simulink model "Induction_Motor_from_B_K_Basu_beautified"  (R2019a)
settings: Solver=FixedStepAuto  StartTime=0.0  StopTime=4  FixedStep=1e-6  RelTol=1e-3
undefined symbols (not defined in the file): sigbuilder_block
libraries: powerlib x14
settings Model: Creator=asus  LastModifiedBy=asus

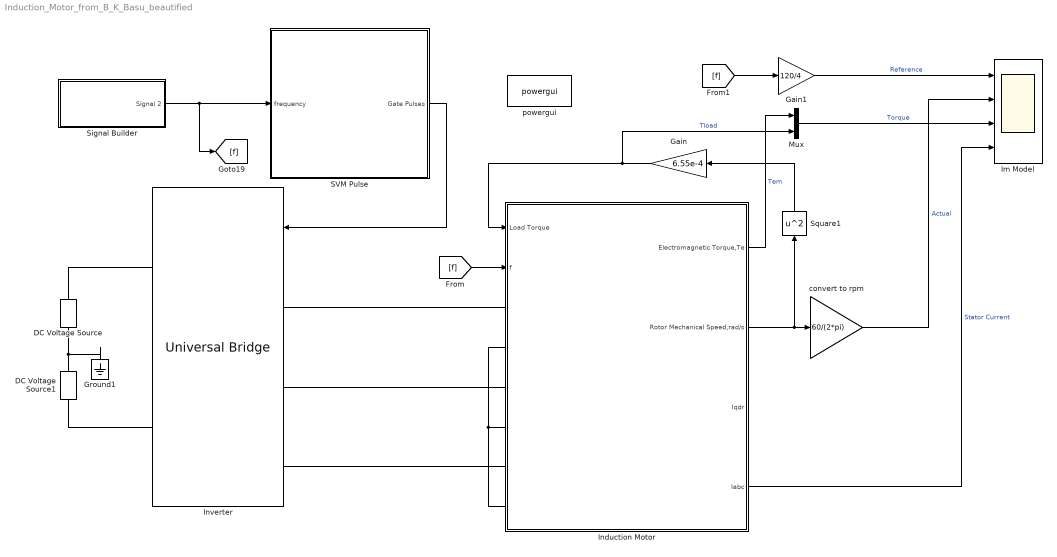
== system Induction_Motor_from_B_K_Basu_beautified ==
  DC Voltage Source : powerlib/Electrical Sources/DC Voltage Source  Amplitude=200  Measurements=None
      settings: SourceProductName=Simscape Electrical
  DC Voltage Source1 : powerlib/Electrical Sources/DC Voltage Source  Amplitude=200  Measurements=None
      settings: SourceProductName=Simscape Electrical
  Gain : Gain  Gain=6.55e-4
  Gain1 : Gain  Gain=120/4
  Ground1 : powerlib/Elements/Ground  LConnTagsString=a
      settings: SourceProductName=Simscape Electrical
  Im Model : Scope  NumInputPorts=4
  Induction Motor : Subsystem  mask{fb=50, Rs=0.603, Rr=0.7, Lls=3.20538e-3, Llr=2.93227e-3, Lm=.0749938, p=4, J=.031, D=.00114}
      mask prompts: fb "Base Frequency. Hz"; Rs "Stator Resistance, Rs"; Rr "Rotor Resistamce, Rr"; Lls "Stator Leakage inductance, Lls"; Llr "Rotor Leakage inductance, Llr"; Lm "Magnetizing Inductance,Lm"; p "Actual Number of Pole,P"; J "Inertia, J"; D "Damping Coefficient,D(Nms)"
      mask help:
      | Frequency is your actual excitation frequency. Base frequency is the maximum frequency for the drive.
      | This are initialized.
      | we=2*pi*f;
      | wb=2*pi*fb;
      | xls=wb*Lls;
      | xlr=wb*Llr;
      | xmeg=wb*Lm;
      | xm=1/(1/xls+1/xlr+1/xmeg);
      mask init:
      | wb=2*pi*fb;
      | xls=wb*Lls;
      | xlr=wb*Llr;
      | xmeg=wb*Lm;
      | xm=1/(1/xls+1/xlr+1/xmeg);
      mask Help:
      | Frequency, f=input from user
      | Base Frequency, fb= input from user
      | Rotor Resistamce= Rr
      | Stator Resistamce= Rs
      | Stator Leakage inductance=Lls
      | Rotor Leakage inductance= Llr
      | Magnetizing Inductance=Lm
      | Actual Number of Pole=p
      | Inertia= J
  Inverter : powerlib/Power Electronics/Universal Bridge  Arms=3  SnubberResistance=1e5  SnubberCapacitance=inf  Device=IGBT / Diodes  Ron=1e-3  Lon=0  ForwardVoltages="[  0  0  ]"  ForwardVoltage=0  GTOparameters=[ 10e-6 , 20e-6 ]  IGBTparameters=[ 1e-6 , 2e-6 ]  Measurements=None  Measurements_2=None  converterType=Rectifier
      settings: SourceProductName=Simscape Electrical
  Mux : Mux  Inputs=2
  SVM Pulse : Subsystem
  Signal Builder : Subsystem  Tag=STV Subsys  LoadFcn=sigbuilder_block('load');  StartFcn=sigbuilder_block('start');  StopFcn=sigbuilder_block('stop');  ClipboardFcn=sigbuilder_block('clipboard');  mask(Sigbuilder block){tuvar=[0:10]}
      mask help: Simulink:masks:SigbuilderBlock_MD
      mask init:
      | if ~strcmp(get_param(bdroot(gcbh),'SimulationStatus'),'stopped') tuvar = sigbuilder_block('maskInit'); end
      settings: CopyFcn=sigbuilder_block('copy');  DeleteFcn=sigbuilder_block('delete');  ModelCloseFcn=sigbuilder_block('modelClose');  PreSaveFcn=sigbuilder_block('preSave');  PauseFcn=sigbuilder_block('pause');  ContinueFcn=sigbuilder_block('continue');  NameChangeFcn=sigbuilder_block('namechange');  OpenFcn=sigbuilder_block('open',[0 30 960 455.4 ]);  CloseFcn=sigbuilder_block('close');
      mask Display: plot(0, 0, 100, 100,[2, 2, 32, 32, 2], [68, 8, 8, 68, 68],[32, 2], [38, 38], [32, 19, 2],[53, 60, 44], [32, 17, 17, 2],[16, 16, 31, 31]);txt = getActiveGroup(gcbh);text(2, 100, txt,'verticalAlignment', 'top');
  Square1 : Math  Operator=square  SaturateOnIntegerOverflow=on
  convert to rpm : Gain  Gain=60/(2*pi)
  powergui : powerlib/powergui  Priority=1  SimulationMode=Discrete  SampleTime=1e-6  frequency=60  Iterations=50  frequencyindice=0  Pbase=100e6  ErrMax=1e-4  UnitsV=kV  UnitsW=MW  buscounter=0  FunctionMessages=off  echomessages=off  EnableUseOfTLC=off  CurrentSourceSwitches=off  DisableSnubberDevices=off  DisableRonSwitches=off  DisableVfSwitches=off  DisplayEquations=off  AutomaticDiscreteSolvers=off  SolverType=Tustin/Backward Euler (TBE)  Interpol=off  ExternalGateDelay=off  methode=off  Ts=100  x0status=blocks  SPID=on  SwTol=0  HookPort=off  NonlinearTolerance=0  nMaxIteration=15  ContinueOnMaxIteration=off  RestoreLinks=warning  ResistiveCurrentMeasurement=off  Frange=[0:2:500]  Ylog=off  Xlog=on  ShowGrid=off  save=off  variable=ZData  structure=0  ZoomFFT=off  StartTime=0.0  cycles=1  DisplayStyle=1  fundamental=60  FreqAxis=off  MaxFrequency=1000  frequencyindicesteady=1  RmsSteady=1  display=off
      settings: SourceProductName=Simscape Electrical
  wires:
  Signal Builder/1(Signal 2) -> [f], SVM Pulse/1(frequency)
  Induction Motor/1(" Electromagnetic Torque,Te ") -> Mux/1  "Tem"
  Induction Motor/2(" Rotor Mechanical Speed,rad/s ") -> Square1/1, convert to rpm/1
  Square1/1 -> Gain/1
  convert to rpm/1 -> Im Model/2  "Actual"
  Gain/1 -> Induction Motor/1(Load Torque), Mux/2  "Tload"
  SVM Pulse/1(Gate Pulses) -> Inverter/1
  [f] -> Induction Motor/2("f ")
  [f] -> Gain1/1
  Gain1/1 -> Im Model/1  "Reference"
  Mux/1 -> Im Model/3  "Torque"
  Induction Motor/4("      Iabc    ") -> Im Model/4  "Stator Current"
  connections:
  Induction Motor/LConn4 -- Induction Motor/LConn2 -- Induction Motor/LConn6
  DC Voltage Source1/RConn1 -- Ground1/LConn1 -- DC Voltage Source/LConn1
  DC Voltage Source1/LConn1 -- Inverter/RConn2
  DC Voltage Source/RConn1 -- Inverter/RConn1
  Inverter/LConn1 -- Induction Motor/LConn1
  Inverter/LConn2 -- Induction Motor/LConn3
  Inverter/LConn3 -- Induction Motor/LConn5

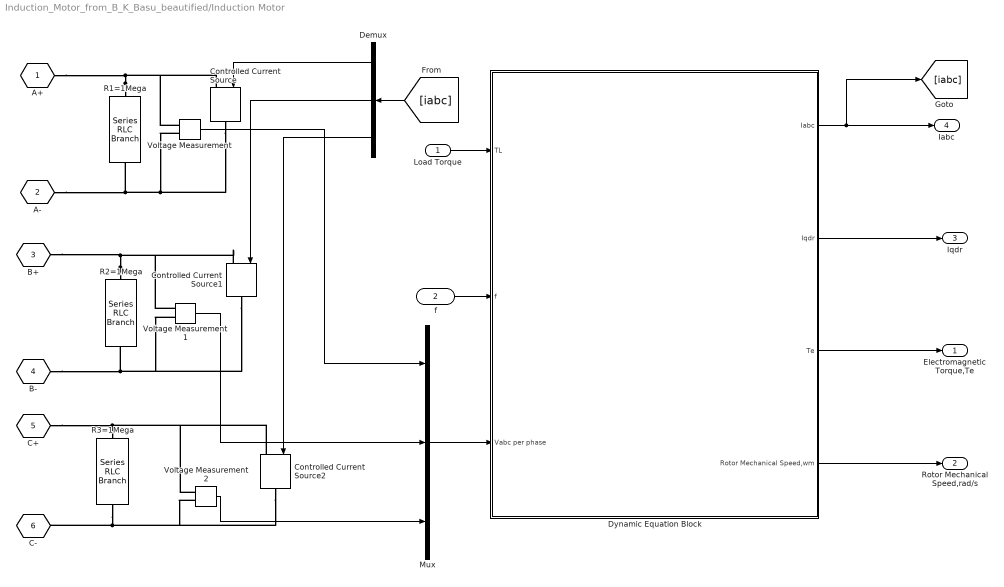
== system Induction_Motor_from_B_K_Basu_beautified/Induction Motor ==
  Load Torque : Inport
  "f " : Inport  Port=2
  Controlled Current Source : powerlib/Electrical Sources/Controlled Current Source  Initialize=on  Source_Type=AC  Amplitude=0  Phase=0  Frequency=0  Measurements=None
      settings: SourceProductName=Simscape Electrical
  Controlled Current Source1 : powerlib/Electrical Sources/Controlled Current Source  Initialize=on  Source_Type=AC  Amplitude=0  Phase=0  Frequency=0  Measurements=None
      settings: SourceProductName=Simscape Electrical
  Controlled Current Source2 : powerlib/Electrical Sources/Controlled Current Source  Initialize=on  Source_Type=AC  Amplitude=0  Phase=0  Frequency=0  Measurements=None
      settings: SourceProductName=Simscape Electrical
  Demux : Demux  Outputs=3
  Dynamic Equation Block : Subsystem
  Mux : Mux  Inputs=3
  R1=1Mega : powerlib/Elements/Series RLC Branch  LConnTagsString=__new0  RConnTagsString=__new0  BranchType=R  Resistance=1e6  Inductance=1e-3  SetiL0=off  InitialCurrent=0  Capacitance=1e-6  Setx0=off  InitialVoltage=0  Measurements=None
      settings: SourceProductName=Simscape Electrical
  R2=1Mega : powerlib/Elements/Series RLC Branch  LConnTagsString=__new0  RConnTagsString=__new0  BranchType=R  Resistance=1e6  Inductance=1e-3  SetiL0=off  InitialCurrent=0  Capacitance=1e-6  Setx0=off  InitialVoltage=0  Measurements=None
      settings: SourceProductName=Simscape Electrical
  R3=1Mega : powerlib/Elements/Series RLC Branch  LConnTagsString=__new0  RConnTagsString=__new0  BranchType=R  Resistance=1e6  Inductance=1e-3  SetiL0=off  InitialCurrent=0  Capacitance=1e-6  Setx0=off  InitialVoltage=0  Measurements=None
      settings: SourceProductName=Simscape Electrical
  Voltage Measurement : powerlib/Measurements/Voltage Measurement  PhasorSimulation=off  OutputType=Complex  PSBequivalent=0
      settings: SourceProductName=Simscape Electrical
  Voltage Measurement1 : powerlib/Measurements/Voltage Measurement  PhasorSimulation=off  OutputType=Complex  PSBequivalent=0
      settings: SourceProductName=Simscape Electrical
  Voltage Measurement2 : powerlib/Measurements/Voltage Measurement  PhasorSimulation=off  OutputType=Complex  PSBequivalent=0
      settings: SourceProductName=Simscape Electrical
  A+ : PMIOPort  Tag=PMCPort  Side=Left
  A- : PMIOPort  Tag=PMCPort  Port=2  Side=Left
  B+ : PMIOPort  Tag=PMCPort  Port=3  Side=Left
  B- : PMIOPort  Tag=PMCPort  Port=4  Side=Left
  C+ : PMIOPort  Tag=PMCPort  Port=5  Side=Left
  C- : PMIOPort  Tag=PMCPort  Port=6  Side=Left
  " Electromagnetic Torque,Te " : Outport
  " Rotor Mechanical Speed,rad/s " : Outport  Port=2
  " Iqdr     " : Outport  Port=3
  "      Iabc    " : Outport  Port=4
  wires:
  Dynamic Equation Block/4("Rotor Mechanical Speed,wm ") -> " Rotor Mechanical Speed,rad/s "/1
  Voltage Measurement/1 -> Mux/1
  Load Torque/1 -> Dynamic Equation Block/1(TL)
  Voltage Measurement1/1 -> Mux/2
  Voltage Measurement2/1 -> Mux/3
  Mux/1 -> Dynamic Equation Block/3(Vabc per phase)
  Dynamic Equation Block/3(Te) -> " Electromagnetic Torque,Te "/1
  Dynamic Equation Block/1(Iabc) -> [iabc], "      Iabc    "/1
  Dynamic Equation Block/2("Iqdr ") -> " Iqdr     "/1
  [iabc] -> Demux/1
  Demux/1 -> Controlled Current Source/1
  Demux/2 -> Controlled Current Source1/1
  Demux/3 -> Controlled Current Source2/1
  "f "/1 -> Dynamic Equation Block/2(f)
  connections:
  Controlled Current Source1/RConn1 -- Voltage Measurement1/LConn2 -- B-/RConn1 -- R2=1Mega/RConn1
  R2=1Mega/LConn1 -- Controlled Current Source1/LConn1 -- Voltage Measurement1/LConn1 -- B+/RConn1
  R3=1Mega/LConn1 -- Controlled Current Source2/LConn1 -- Voltage Measurement2/LConn1 -- C+/RConn1
  R3=1Mega/RConn1 -- Controlled Current Source2/RConn1 -- Voltage Measurement2/LConn2 -- C-/RConn1
  R1=1Mega/LConn1 -- Voltage Measurement/LConn1 -- Controlled Current Source/LConn1 -- A+/RConn1
  Voltage Measurement/LConn2 -- R1=1Mega/RConn1 -- A-/RConn1 -- Controlled Current Source/RConn1

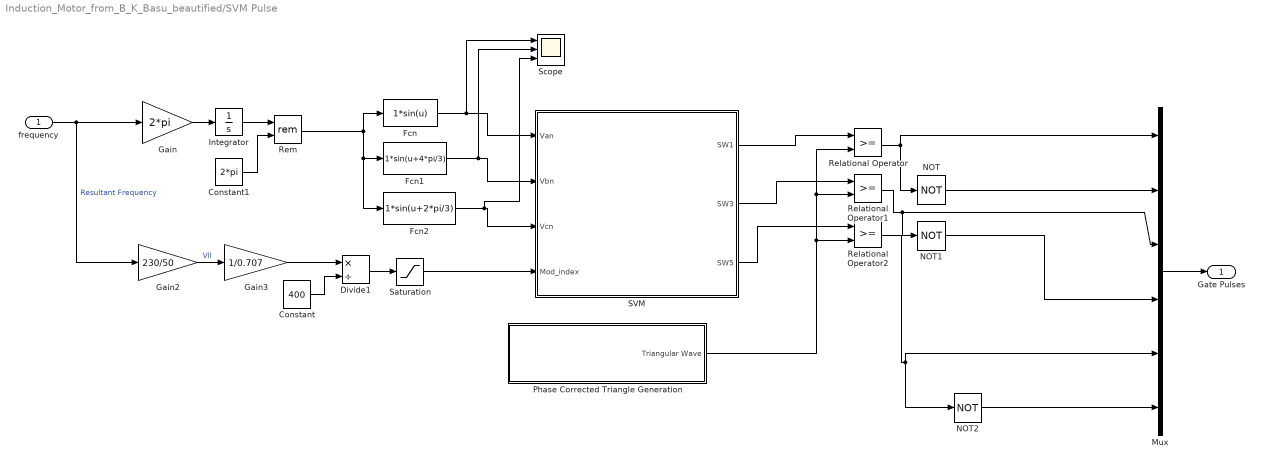
== system Induction_Motor_from_B_K_Basu_beautified/SVM Pulse ==
  frequency : Inport
  Constant : Constant  Value=400
  Constant1 : Constant  Value=2*pi
  Divide1 : Product  Inputs=*/
  Fcn : Fcn  Expr=1*sin(u)
  Fcn1 : Fcn  Expr=1*sin(u+4*pi/3)
  Fcn2 : Fcn  Expr=1*sin(u+2*pi/3)
  Gain : Gain  Gain=2*pi
  Gain2 : Gain  Gain=230/50
  Gain3 : Gain  Gain=1/0.707
  Integrator : Integrator
  Mux : Mux  Inputs=6
  NOT : Logic  Operator=NOT  IconShape=distinctive  AllPortsSameDT=off  OutDataTypeStr=boolean
  NOT1 : Logic  Operator=NOT  IconShape=distinctive  AllPortsSameDT=off  OutDataTypeStr=boolean
  NOT2 : Logic  Operator=NOT  IconShape=distinctive  AllPortsSameDT=off  OutDataTypeStr=boolean
  Phase Corrected Triangle Generation : Subsystem
  Relational Operator : RelationalOperator  OutDataTypeStr=boolean  RndMeth=Nearest
  Relational Operator1 : RelationalOperator  OutDataTypeStr=boolean  RndMeth=Nearest
  Relational Operator2 : RelationalOperator  OutDataTypeStr=boolean  RndMeth=Nearest
  Rem : Math  Operator=rem  SaturateOnIntegerOverflow=on
  SVM : Subsystem
  Saturation : Saturate  UpperLimit=1  LowerLimit=0
  Scope : Scope  NumInputPorts=3
  Gate Pulses : Outport
  wires:
  Phase Corrected Triangle Generation/1(Triangular Wave) -> Relational Operator/2, Relational Operator1/2, Relational Operator2/2
  SVM/3(SW5) -> Relational Operator2/1
  NOT/1 -> Mux/2
  Relational Operator2/1 -> Mux/5, NOT2/1
  Relational Operator1/1 -> NOT1/1, Mux/3
  SVM/1(SW1) -> Relational Operator/1
  SVM/2(SW3) -> Relational Operator1/1
  NOT2/1 -> Mux/6
  Saturation/1 -> SVM/4(Mod_index)
  Relational Operator/1 -> Mux/1, NOT/1
  NOT1/1 -> Mux/4
  Mux/1 -> Gate Pulses/1
  Rem/1 -> Fcn/1, Fcn2/1, Fcn1/1
  Fcn/1 -> Scope/1, SVM/1(Van)
  Fcn1/1 -> Scope/2, SVM/2(Vbn)
  Fcn2/1 -> Scope/3, SVM/3(Vcn)
  Divide1/1 -> Saturation/1
  Gain3/1 -> Divide1/1
  Gain2/1 -> Gain3/1  "Vll"
  frequency/1 -> Gain/1, Gain2/1  "Resultant Frequency"
  Constant/1 -> Divide1/2
  Gain/1 -> Integrator/1
  Integrator/1 -> Rem/1
  Constant1/1 -> Rem/2

== system Induction_Motor_from_B_K_Basu_beautified/Signal Builder ==
  Demux : Demux  Tag=STV Demux  Outputs=1
  FromWs : FromWorkspace  Tag=STV FromWs  VariableName=tuvar  SampleTime=0
      SigBuilderData=|
      | common.afterFinalStr = 'Extrapolate'
      | common.sampleTime = 0
      | dataSet.timeRange = [0 10]
      | dataSet.name = 'Group 1'
      | sbobj.Groups.Name = 'Group 1'
      | sbobj.Groups.Signals.Name = 'Signal 2'
      | sbobj.Groups.Signals.XData = [0 2 3 3 3.5 3.5 4 4 5 10]
      | sbobj.Groups.Signals.YData = [5 50 25 20 20 30 30 10 10 40]
  Signal 2 : Outport  Tag=STV Outport
  wires:
  FromWs/1 -> Demux/1
  Demux/1 -> Signal 2/1

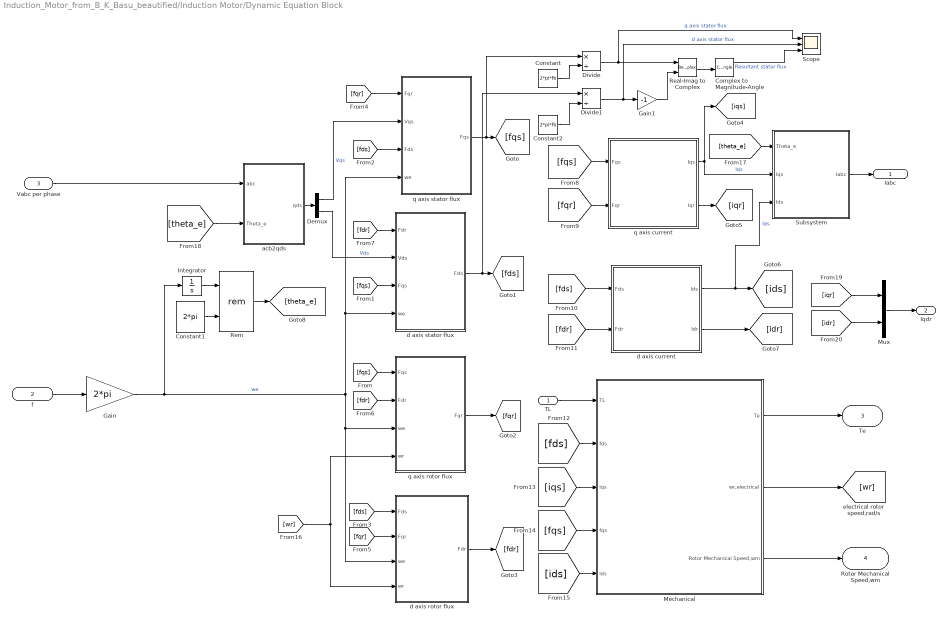
== system Induction_Motor_from_B_K_Basu_beautified/Induction Motor/Dynamic Equation Block ==
  TL : Inport
  f : Inport  Port=2
  Vabc per phase : Inport  Port=3
  Complex to Magnitude-Angle : ComplexToMagnitudeAngle
  Constant : Constant  Value=2*pi*fb
  Constant1 : Constant  Value=2*pi
  Constant2 : Constant  Value=2*pi*fb
  Demux : Demux  Outputs=2
  Divide : Product  Inputs=*/
  Divide1 : Product  Inputs=*/
  Gain : Gain  Gain=2*pi
  Gain1 : Gain  Gain=-1
  Integrator : Integrator
  Mechanical : Subsystem
  Mux : Mux  Inputs=2
  Real-Imag to Complex : RealImagToComplex
  Rem : Math  Operator=rem  SaturateOnIntegerOverflow=on
  Scope : Scope  NumInputPorts=3
  Subsystem : Subsystem
  acb2qds : Subsystem
  d axis current : Subsystem
  d axis rotor flux : Subsystem
  d axis stator flux : Subsystem
  q axis current : Subsystem
  q axis rotor flux : Subsystem
  "q axis stator flux " : Subsystem
  Iabc : Outport
  "Iqdr " : Outport  Port=2
  Te : Outport  Port=3
  "Rotor Mechanical Speed,wm " : Outport  Port=4
  wires:
  "q axis stator flux "/1(Fqs) -> Divide/1, [fqs]
  [fqr] -> "q axis stator flux "/1(Fqr)
  Gain/1 -> d axis rotor flux/3("we "), q axis rotor flux/3("we "), d axis stator flux/4(we), "q axis stator flux "/4(we), Integrator/1  "we"
  [fds] -> "q axis stator flux "/3(Fds)
  [wr] -> d axis rotor flux/4(wr), q axis rotor flux/4(wr)
  Demux/2 -> d axis stator flux/2(Vds)  "Vds"
  d axis rotor flux/1(Fdr) -> [fdr]
  [fds] -> d axis rotor flux/1("Fds  ")
  q axis current/2(Iqr) -> [iqr]
  [fds] -> d axis current/1(Fds)
  [fdr] -> d axis current/2(Fdr)
  [fqs] -> q axis current/1(Fqs)
  q axis current/1(Iqs) -> [iqs], Subsystem/2(Iqs)  "Iqs"
  d axis stator flux/1(Fds) -> Divide1/1, [fds]
  [fqr] -> q axis current/2(Fqr)
  q axis rotor flux/1(Fqr) -> [fqr]
  [fdr] -> d axis stator flux/1("Fdr ")
  [fqs] -> q axis rotor flux/1("Fqs  ")
  [fdr] -> q axis rotor flux/2("Fdr ")
  [fqs] -> d axis stator flux/3("Fqs ")
  [fqr] -> d axis rotor flux/2("Fqr  ")
  d axis current/1(Ids) -> [ids], Subsystem/3(Ids)  "Ids"
  Demux/1 -> "q axis stator flux "/2(Vqs)  "Vqs"
  d axis current/2(Idr) -> [idr]
  acb2qds/1(qds) -> Demux/1
  TL/1 -> Mechanical/1(TL)
  Mechanical/1(Te) -> Te/1
  Mechanical/2(wr,electrical) -> [wr]
  Mechanical/3("Rotor Mechanical Speed,wm ") -> "Rotor Mechanical Speed,wm "/1
  [fds] -> Mechanical/2(fds)
  [iqs] -> Mechanical/3(iqs)
  [fqs] -> Mechanical/4(fqs)
  [ids] -> Mechanical/5(ids)
  Vabc per phase/1 -> acb2qds/1(abc)
  Integrator/1 -> Rem/1
  Constant1/1 -> Rem/2
  Rem/1 -> [theta_e]
  Subsystem/1(Iabc) -> Iabc/1
  [theta_e] -> Subsystem/1(Theta_e)
  [theta_e] -> acb2qds/2(Theta_e)
  [iqr] -> Mux/1
  [idr] -> Mux/2
  Mux/1 -> "Iqdr "/1
  f/1 -> Gain/1
  Constant/1 -> Divide/2
  Constant2/1 -> Divide1/2
  Divide1/1 -> Scope/2, Gain1/1  "d axis stator flux"
  Divide/1 -> Scope/1, Real-Imag to Complex/1  "q axis stator flux"
  Gain1/1 -> Real-Imag to Complex/2
  Real-Imag to Complex/1 -> Complex to Magnitude-Angle/1
  Complex to Magnitude-Angle/1 -> Scope/3  "Resultant stator flux"

== system Induction_Motor_from_B_K_Basu_beautified/SVM Pulse/Phase Corrected Triangle Generation ==
  Constant : Constant
  Gain : Gain  Gain=2*5000
  Integrator : Integrator
  Pulse Generator : DiscretePulseGenerator  PulseType=Time based  Amplitude=2  Period=1/5000  PulseWidth=50
  Sum : Sum  Inputs=|+-
  Triangular Wave : Outport
  wires:
  Gain/1 -> Triangular Wave/1
  Pulse Generator/1 -> Sum/1
  Sum/1 -> Integrator/1
  Integrator/1 -> Gain/1
  Constant/1 -> Sum/2

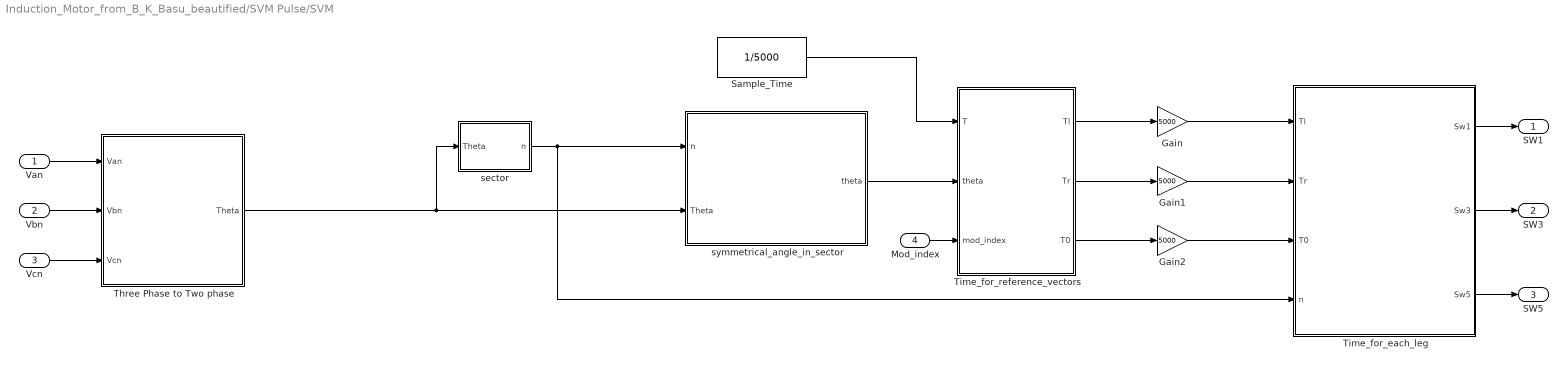
== system Induction_Motor_from_B_K_Basu_beautified/SVM Pulse/SVM ==
  Van : Inport
  Vbn : Inport  Port=2
  Vcn : Inport  Port=3
  Mod_index : Inport  Port=4
  Gain : Gain  Gain=5000
  Gain1 : Gain  Gain=5000
  Gain2 : Gain  Gain=5000
  Sample_Time : Constant  Value=1/5000
  "Three Phase to Two phase " : MATLAB Function  TreatAsAtomicUnit=on
  Time_for_each_leg : MATLAB Function  TreatAsAtomicUnit=on
  Time_for_reference_vectors : MATLAB Function  TreatAsAtomicUnit=on
  "sector " : MATLAB Function  TreatAsAtomicUnit=on
  symmetrical_angle_in_sector : MATLAB Function  TreatAsAtomicUnit=on
  SW1 : Outport
  SW3 : Outport  Port=2
  SW5 : Outport  Port=3
  wires:
  Sample_Time/1 -> Time_for_reference_vectors/1(T)
  Time_for_reference_vectors/2(Tr) -> Gain1/1
  Time_for_reference_vectors/1(Tl) -> Gain/1
  Time_for_reference_vectors/3(T0) -> Gain2/1
  symmetrical_angle_in_sector/1(theta) -> Time_for_reference_vectors/2(theta)
  "Three Phase to Two phase "/1(Theta) -> symmetrical_angle_in_sector/2(Theta), "sector "/1(Theta)
  Vbn/1 -> "Three Phase to Two phase "/2(Vbn)
  Vcn/1 -> "Three Phase to Two phase "/3(Vcn)
  Van/1 -> "Three Phase to Two phase "/1(Van)
  Gain/1 -> Time_for_each_leg/1(Tl)
  Gain1/1 -> Time_for_each_leg/2(Tr)
  Gain2/1 -> Time_for_each_leg/3(T0)
  "sector "/1(n) -> Time_for_each_leg/4(n), symmetrical_angle_in_sector/1(n)
  Time_for_each_leg/1(Sw1) -> SW1/1
  Time_for_each_leg/2(Sw3) -> SW3/1
  Time_for_each_leg/3(Sw5) -> SW5/1
  Mod_index/1 -> Time_for_reference_vectors/3(mod_index)

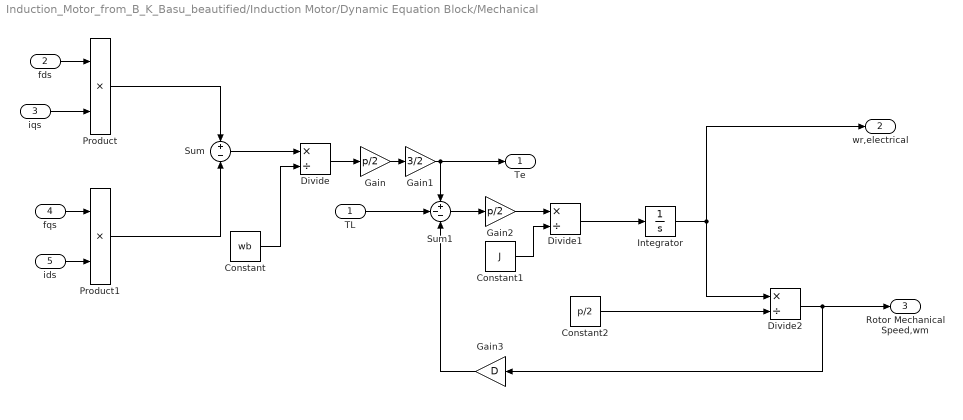
== system Induction_Motor_from_B_K_Basu_beautified/Induction Motor/Dynamic Equation Block/Mechanical ==
  TL : Inport
  fds : Inport  Port=2
  iqs : Inport  Port=3
  fqs : Inport  Port=4
  ids : Inport  Port=5
  Constant : Constant  Value=wb
  Constant1 : Constant  Value=J
  Constant2 : Constant  Value=p/2
  Divide : Product  Inputs=*/
  Divide1 : Product  Inputs=*/
  Divide2 : Product  Inputs=*/
  Gain : Gain  Gain=p/2
  Gain1 : Gain  Gain=3/2
  Gain2 : Gain  Gain=p/2
  Gain3 : Gain  Gain=D
  Integrator : Integrator
  Product : Product
  Product1 : Product
  Sum : Sum  Inputs=+-
  Sum1 : Sum  Inputs=+--
  Te : Outport
  wr,electrical : Outport  Port=2
  "Rotor Mechanical Speed,wm " : Outport  Port=3
  wires:
  Sum1/1 -> Gain2/1
  Product/1 -> Sum/1
  Divide1/1 -> Integrator/1
  Constant2/1 -> Divide2/2
  Constant1/1 -> Divide1/2
  Sum/1 -> Divide/1
  Gain1/1 -> Te/1, Sum1/1
  TL/1 -> Sum1/2
  Divide2/1 -> Gain3/1, "Rotor Mechanical Speed,wm "/1
  Gain/1 -> Gain1/1
  Constant/1 -> Divide/2
  Gain2/1 -> Divide1/1
  Product1/1 -> Sum/2
  Divide/1 -> Gain/1
  fds/1 -> Product/1
  ids/1 -> Product1/2
  fqs/1 -> Product1/1
  iqs/1 -> Product/2
  Integrator/1 -> Divide2/1, wr,electrical/1
  Gain3/1 -> Sum1/3

== system Induction_Motor_from_B_K_Basu_beautified/Induction Motor/Dynamic Equation Block/Subsystem ==
  Theta_e : Inport
  Iqs : Inport  Port=2
  Ids : Inport  Port=3
  Fcn : Fcn  Expr=(u(2)*cos(u(1)))+(u(3)*sin(u(1)))
  Fcn1 : Fcn  Expr=(-u(2)*sin(u(1)))+(u(3)*cos(u(1)))
  Fcn2 : Fcn  Expr=u(1)
  Fcn3 : Fcn  Expr=(-u(1)*1/2)+(-sqrt(3)/2*u(2))
  Fcn4 : Fcn  Expr=(-u(1)*1/2)+(sqrt(3)/2*u(2))
  Mux : Mux  Inputs=3
  Mux1 : Mux  Inputs=2
  Mux2 : Mux  Inputs=3
  Iabc : Outport
  wires:
  Fcn3/1 -> Mux2/2
  Fcn/1 -> Mux1/1  "Iqs"
  Mux1/1 -> Fcn4/1, Fcn3/1, Fcn2/1
  Mux/1 -> Fcn1/1, Fcn/1
  Fcn1/1 -> Mux1/2  "Ids"
  Iqs/1 -> Mux/2
  Fcn2/1 -> Mux2/1
  Fcn4/1 -> Mux2/3
  Mux2/1 -> Iabc/1
  Theta_e/1 -> Mux/1
  Ids/1 -> Mux/3

== system Induction_Motor_from_B_K_Basu_beautified/Induction Motor/Dynamic Equation Block/acb2qds ==
  abc : Inport
  Theta_e : Inport  Port=2
  Fcn : Fcn  Expr=u(1)
  Fcn1 : Fcn  Expr=(-u(2)+u(3))/sqrt(3)
  Fcn2 : Fcn  Expr=(u(1)*cos(u(3)))-(u(2)*sin(u(3)))
  Fcn3 : Fcn  Expr=(u(1)*sin(u(3)))+(u(2)*cos(u(3)))
  Mux1 : Mux  Inputs=2
  Mux2 : Mux  Inputs=3
  qds : Outport
  wires:
  Fcn1/1 -> Mux2/2  "Vdstator"
  abc/1 -> Fcn1/1, Fcn/1
  Mux2/1 -> Fcn3/1, Fcn2/1
  Theta_e/1 -> Mux2/3
  Fcn2/1 -> Mux1/1  "Vqs"
  Fcn3/1 -> Mux1/2  "Vds"
  Mux1/1 -> qds/1
  Fcn/1 -> Mux2/1  "Vqstator"

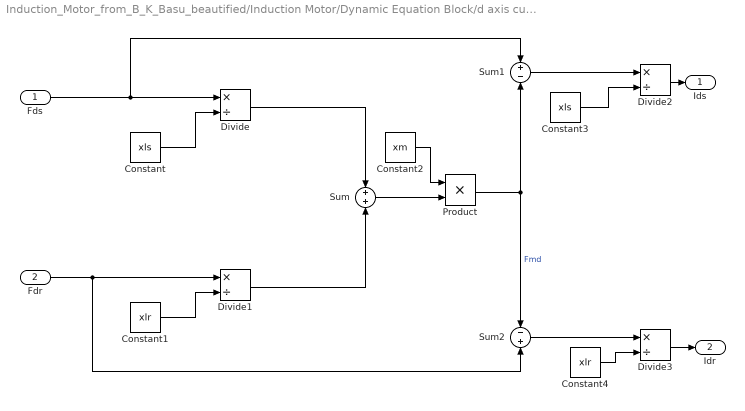
== system Induction_Motor_from_B_K_Basu_beautified/Induction Motor/Dynamic Equation Block/d axis current ==
  Fds : Inport
  Fdr : Inport  Port=2
  Constant : Constant  Value=xls
  Constant1 : Constant  Value=xlr
  Constant2 : Constant  Value=xm
  Constant3 : Constant  Value=xls
  Constant4 : Constant  Value=xlr
  Divide{,1..3} (4 alike) : Product  Inputs=*/
  Product : Product
  Sum : Sum
  Sum1 : Sum  Inputs=+-
  Sum2 : Sum  Inputs=-+
  Ids : Outport
  Idr : Outport  Port=2
  wires:
  Fdr/1 -> Sum2/2, Divide1/1
  Constant2/1 -> Product/1
  Product/1 -> Sum2/1, Sum1/2  "Fmd"
  Constant/1 -> Divide/2
  Sum/1 -> Product/2
  Divide1/1 -> Sum/2
  Constant1/1 -> Divide1/2
  Fds/1 -> Sum1/1, Divide/1
  Divide/1 -> Sum/1
  Sum1/1 -> Divide2/1
  Constant3/1 -> Divide2/2
  Divide2/1 -> Ids/1
  Sum2/1 -> Divide3/1
  Constant4/1 -> Divide3/2
  Divide3/1 -> Idr/1

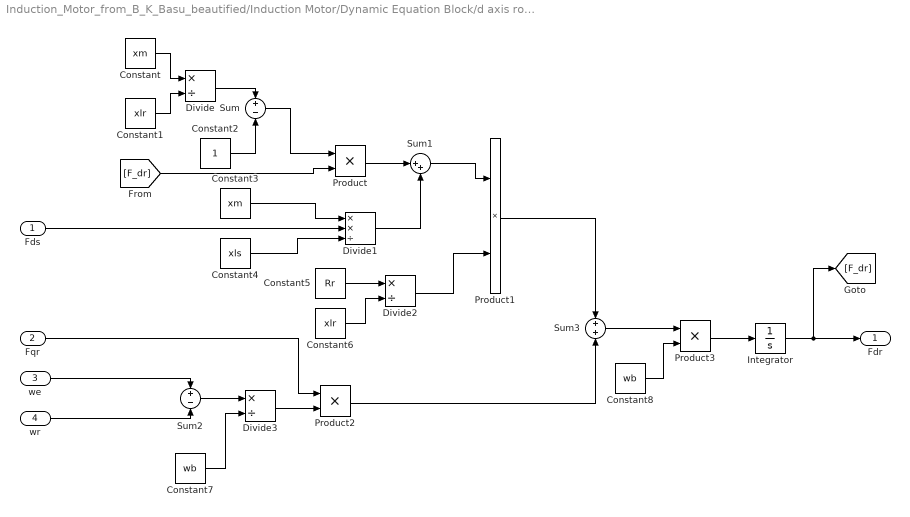
== system Induction_Motor_from_B_K_Basu_beautified/Induction Motor/Dynamic Equation Block/d axis rotor flux ==
  "Fds  " : Inport
  "Fqr  " : Inport  Port=2
  "we " : Inport  Port=3
  wr : Inport  Port=4
  Constant : Constant  Value=xm
  Constant1 : Constant  Value=xlr
  Constant2 : Constant
  Constant3 : Constant  Value=xm
  Constant4 : Constant  Value=xls
  Constant5 : Constant  Value=Rr
  Constant6 : Constant  Value=xlr
  Constant7 : Constant  Value=wb
  Constant8 : Constant  Value=wb
  Divide : Product  Inputs=*/
  Divide1 : Product  Inputs=**/
  Divide2 : Product  Inputs=*/
  Divide3 : Product  Inputs=*/
  Integrator : Integrator
  Product{,1..3} (4 alike) : Product
  Sum : Sum  Inputs=+-
  Sum1 : Sum  Inputs=|++
  Sum2 : Sum  Inputs=+-
  Sum3 : Sum
  Fdr : Outport
  wires:
  Constant2/1 -> Sum/2
  Sum/1 -> Product/1
  Constant/1 -> Divide/1
  Constant3/1 -> Divide1/1
  Sum3/1 -> Product3/1
  "Fds  "/1 -> Divide1/2
  Constant4/1 -> Divide1/3
  [F_dr] -> Product/2
  Divide1/1 -> Sum1/2
  Constant1/1 -> Divide/2
  Product3/1 -> Integrator/1
  Divide/1 -> Sum/1
  Constant5/1 -> Divide2/1
  Constant7/1 -> Divide3/2
  wr/1 -> Sum2/2
  Constant8/1 -> Product3/2
  Product2/1 -> Sum3/2
  "Fqr  "/1 -> Product2/1
  Product/1 -> Sum1/1
  Sum1/1 -> Product1/1
  "we "/1 -> Sum2/1
  Integrator/1 -> [F_dr], Fdr/1
  Sum2/1 -> Divide3/1
  Product1/1 -> Sum3/1
  Divide3/1 -> Product2/2
  Divide2/1 -> Product1/2
  Constant6/1 -> Divide2/2

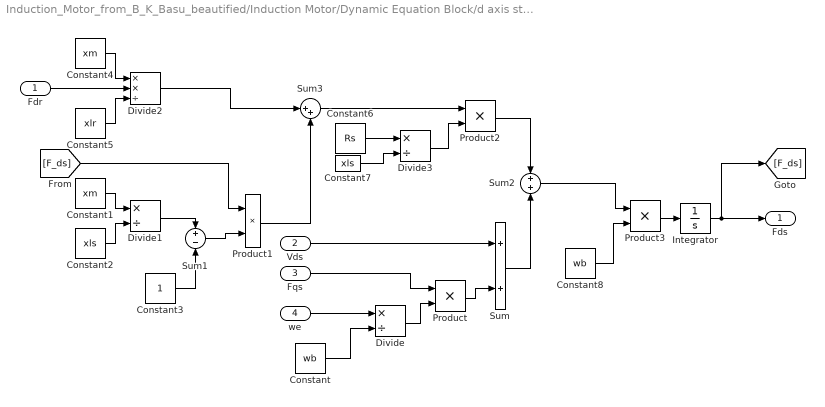
== system Induction_Motor_from_B_K_Basu_beautified/Induction Motor/Dynamic Equation Block/d axis stator flux ==
  "Fdr " : Inport
  Vds : Inport  Port=2
  "Fqs " : Inport  Port=3
  we : Inport  Port=4
  Constant : Constant  Value=wb
  Constant1 : Constant  Value=xm
  Constant2 : Constant  Value=xls
  Constant3 : Constant
  Constant4 : Constant  Value=xm
  Constant5 : Constant  Value=xlr
  Constant6 : Constant  Value=Rs
  Constant7 : Constant  Value=xls
  Constant8 : Constant  Value=wb
  Divide : Product  Inputs=*/
  Divide1 : Product  Inputs=*/
  Divide2 : Product  Inputs=**/
  Divide3 : Product  Inputs=*/
  Integrator : Integrator
  Product{,1..3} (4 alike) : Product
  Sum : Sum
  Sum1 : Sum  Inputs=+-
  Sum2 : Sum
  Sum3 : Sum  Inputs=|++
  Fds : Outport
  wires:
  Constant8/1 -> Product3/2
  "Fdr "/1 -> Divide2/2
  Product2/1 -> Sum2/1
  Vds/1 -> Sum/1
  Divide3/1 -> Product2/2
  Constant7/1 -> Divide3/2
  Constant6/1 -> Divide3/1
  Sum3/1 -> Product2/1
  Product1/1 -> Sum3/2
  Divide2/1 -> Sum3/1
  Constant2/1 -> Divide1/2
  Sum/1 -> Sum2/2
  Constant1/1 -> Divide1/1
  we/1 -> Divide/1
  Product/1 -> Sum/2
  Constant3/1 -> Sum1/2
  Sum1/1 -> Product1/2
  "Fqs "/1 -> Product/1
  Constant/1 -> Divide/2
  Constant5/1 -> Divide2/3
  Divide/1 -> Product/2
  Sum2/1 -> Product3/1
  Divide1/1 -> Sum1/1
  [F_ds] -> Product1/1
  Constant4/1 -> Divide2/1
  Product3/1 -> Integrator/1
  Integrator/1 -> Fds/1, [F_ds]

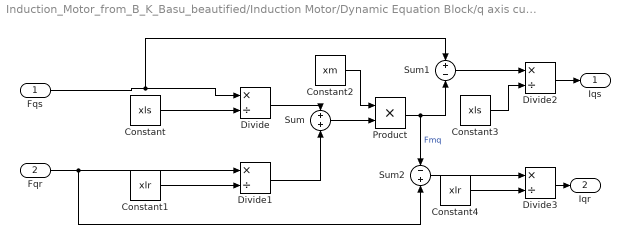
== system Induction_Motor_from_B_K_Basu_beautified/Induction Motor/Dynamic Equation Block/q axis current ==
  Fqs : Inport
  Fqr : Inport  Port=2
  Constant : Constant  Value=xls
  Constant1 : Constant  Value=xlr
  Constant2 : Constant  Value=xm
  Constant3 : Constant  Value=xls
  Constant4 : Constant  Value=xlr
  Divide{,1..3} (4 alike) : Product  Inputs=*/
  Product : Product
  Sum : Sum
  Sum1 : Sum  Inputs=+-
  Sum2 : Sum  Inputs=-+
  Iqs : Outport
  Iqr : Outport  Port=2
  wires:
  Divide/1 -> Sum/1
  Fqs/1 -> Sum1/1, Divide/1
  Constant1/1 -> Divide1/2
  Divide1/1 -> Sum/2
  Sum/1 -> Product/2
  Constant/1 -> Divide/2
  Constant2/1 -> Product/1
  Fqr/1 -> Sum2/2, Divide1/1
  Product/1 -> Sum1/2, Sum2/1  "Fmq"
  Sum1/1 -> Divide2/1
  Constant3/1 -> Divide2/2
  Divide2/1 -> Iqs/1
  Sum2/1 -> Divide3/1
  Constant4/1 -> Divide3/2
  Divide3/1 -> Iqr/1

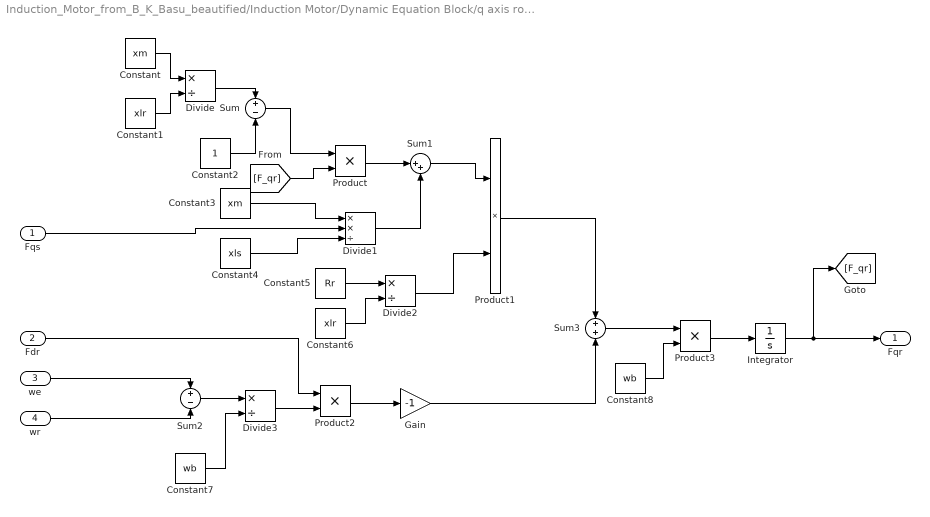
== system Induction_Motor_from_B_K_Basu_beautified/Induction Motor/Dynamic Equation Block/q axis rotor flux ==
  "Fqs  " : Inport
  "Fdr " : Inport  Port=2
  "we " : Inport  Port=3
  wr : Inport  Port=4
  Constant : Constant  Value=xm
  Constant1 : Constant  Value=xlr
  Constant2 : Constant
  Constant3 : Constant  Value=xm
  Constant4 : Constant  Value=xls
  Constant5 : Constant  Value=Rr
  Constant6 : Constant  Value=xlr
  Constant7 : Constant  Value=wb
  Constant8 : Constant  Value=wb
  Divide : Product  Inputs=*/
  Divide1 : Product  Inputs=**/
  Divide2 : Product  Inputs=*/
  Divide3 : Product  Inputs=*/
  Gain : Gain  Gain=-1
  Integrator : Integrator
  Product{,1..3} (4 alike) : Product
  Sum : Sum  Inputs=+-
  Sum1 : Sum  Inputs=|++
  Sum2 : Sum  Inputs=+-
  Sum3 : Sum
  Fqr : Outport
  wires:
  Constant6/1 -> Divide2/2
  Divide2/1 -> Product1/2
  Divide3/1 -> Product2/2
  Product1/1 -> Sum3/1
  Sum2/1 -> Divide3/1
  Integrator/1 -> Fqr/1, [F_qr]
  "we "/1 -> Sum2/1
  Sum1/1 -> Product1/1
  Product2/1 -> Gain/1
  Product/1 -> Sum1/1
  "Fdr "/1 -> Product2/1
  Gain/1 -> Sum3/2
  Constant8/1 -> Product3/2
  wr/1 -> Sum2/2
  Constant7/1 -> Divide3/2
  Constant5/1 -> Divide2/1
  Divide/1 -> Sum/1
  Product3/1 -> Integrator/1
  Constant1/1 -> Divide/2
  Divide1/1 -> Sum1/2
  [F_qr] -> Product/2
  Constant4/1 -> Divide1/3
  "Fqs  "/1 -> Divide1/2
  Sum3/1 -> Product3/1
  Constant3/1 -> Divide1/1
  Constant/1 -> Divide/1
  Sum/1 -> Product/1
  Constant2/1 -> Sum/2

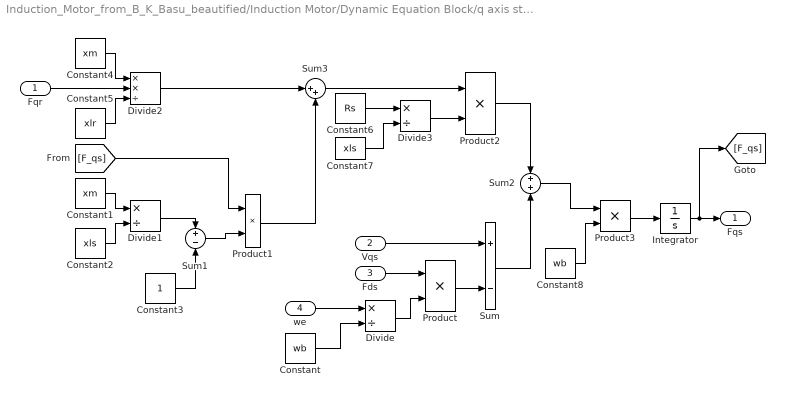
== system Induction_Motor_from_B_K_Basu_beautified/Induction Motor/Dynamic Equation Block/q axis stator flux  ==
  Fqr : Inport
  Vqs : Inport  Port=2
  Fds : Inport  Port=3
  we : Inport  Port=4
  Constant : Constant  Value=wb
  Constant1 : Constant  Value=xm
  Constant2 : Constant  Value=xls
  Constant3 : Constant
  Constant4 : Constant  Value=xm
  Constant5 : Constant  Value=xlr
  Constant6 : Constant  Value=Rs
  Constant7 : Constant  Value=xls
  Constant8 : Constant  Value=wb
  Divide : Product  Inputs=*/
  Divide1 : Product  Inputs=*/
  Divide2 : Product  Inputs=**/
  Divide3 : Product  Inputs=*/
  Integrator : Integrator
  Product{,1..3} (4 alike) : Product
  Sum : Sum  Inputs=+-
  Sum1 : Sum  Inputs=+-
  Sum2 : Sum
  Sum3 : Sum  Inputs=|++
  Fqs : Outport
  wires:
  Constant4/1 -> Divide2/1
  [F_qs] -> Product1/1
  Divide1/1 -> Sum1/1
  Sum2/1 -> Product3/1
  Divide/1 -> Product/2
  Constant5/1 -> Divide2/3
  Constant/1 -> Divide/2
  Fds/1 -> Product/1
  Sum1/1 -> Product1/2
  Constant3/1 -> Sum1/2
  Product/1 -> Sum/2
  we/1 -> Divide/1
  Constant1/1 -> Divide1/1
  Sum/1 -> Sum2/2
  Constant2/1 -> Divide1/2
  Divide2/1 -> Sum3/1
  Product1/1 -> Sum3/2
  Sum3/1 -> Product2/1
  Constant6/1 -> Divide3/1
  Constant7/1 -> Divide3/2
  Divide3/1 -> Product2/2
  Vqs/1 -> Sum/1
  Product2/1 -> Sum2/1
  Fqr/1 -> Divide2/2
  Constant8/1 -> Product3/2
  Product3/1 -> Integrator/1
  Integrator/1 -> Fqs/1, [F_qs]

== matlab function Induction_Motor_from_B_K_Basu_beautified/SVM Pulse/SVM/sector  ==
  data: Theta input; n output
function n = sector(Theta)
%#codegen
n=0;
if (Theta<=pi/3) && (Theta >0)
    n=1;
end
if (Theta<=2*pi/3) && (Theta >pi/3)
    n=2;
end
if (Theta<=pi) && (Theta >2*pi/3)
    n=3;
end
if (Theta<=-2*pi/3) && (Theta >-pi)
    n=4;
end
if (Theta<=-pi/3) && (Theta >-2*pi/3)
    n=5;
end
if (Theta<=0) && (Theta >-pi/3)
    n=6;
end

== matlab function Induction_Motor_from_B_K_Basu_beautified/SVM Pulse/SVM/Three Phase to Two phase  ==
  data: Van input; Vbn input; Vcn input; Theta output
function Theta  = three_to_two_phase(Van,Vbn,Vcn)
%#codegen
Valpha= Van-Vbn/2-Vcn/2;
Vbeta = sqrt(3)/2*(Vbn-Vcn);
Theta = atan2(Vbeta,Valpha);

== matlab function Induction_Motor_from_B_K_Basu_beautified/SVM Pulse/SVM/symmetrical_angle_in_sector ==
  data: n input; Theta input; theta output
function theta = symmetrical_angle_in_sector(n,Theta)
%#codegen
theta=0;
if (n==1)
    theta=Theta;
end
if (n==2)
    theta=Theta-pi/3;
end
if (n==3)
    theta=Theta-2*pi/3;
end
if (n==6)
    theta=pi/3+Theta;
end
if (n==5)
    theta=2*pi/3+Theta;
end
if (n==4)
    theta=pi+Theta;
end

== matlab function Induction_Motor_from_B_K_Basu_beautified/SVM Pulse/SVM/Time_for_reference_vectors ==
  data: Tl output; T input; theta input; Tr output; T0 output; mod_index input
function [Tl,Tr,T0]= Time_for_reference_vectors(T,theta,mod_index)
%#codegen
%a=Vr/Vdc;

%Tr=T*a*(sin(pi/3-theta)/sin(pi/3));
Tr=T*mod_index*sin(pi/3-theta);
% Tl=T*a*sin(theta)/sin(pi/3);
Tl=T*mod_index*sin(theta);
T0=T-Tl-Tr;

== matlab function Induction_Motor_from_B_K_Basu_beautified/SVM Pulse/SVM/Time_for_each_leg ==
  data: Tl input; Sw1 output; Tr input; T0 input; n input; Sw3 output; Sw5 output
function [Sw1,Sw3,Sw5]= Time_for_each_leg(Tl,Tr,T0,n)

%#codegen
Sw1=0;
Sw3=0;
Sw5=0;
if (n==1)
Sw1=Tl+Tr+T0/2;
Sw3=Tl+T0/2;
Sw5=T0/2;
end
if (n==2)
Sw1=Tr+T0/2;
Sw3=Tl+Tr+T0/2;
Sw5=T0/2;
end
if (n==3)
Sw1=T0/2;
Sw3=Tr+Tl+T0/2;
Sw5=Tl+T0/2;
end
if (n==4)
Sw1=T0/2;
Sw3=Tr+T0/2;
Sw5=Tr+Tl+T0/2;
end
if (n==5)
Sw1=Tl+T0/2;
Sw3=T0/2;
Sw5=Tr+Tl+T0/2;
end
if (n==6)
Sw1=Tl+Tr+T0/2;
Sw3=T0/2;
Sw5=Tr+T0/2;
end
